simulink model "PPRZ2l"  (R2016b)
settings: Solver=VariableStepAuto  StartTime=0.0  StopTime=10.0  RelTol=1e-3
settings Model: Creator=kkajak  LastModifiedBy=Karl

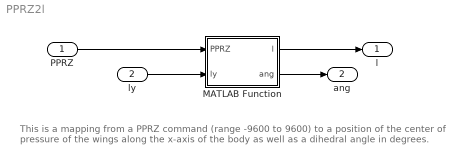
== system PPRZ2l ==
  note: This is a mapping from a PPRZ command (range -9600 to 9600) to a position of the center
      | of pressure of the wings along the x-axis of the body as well as a dihedral angle in degrees.
  PPRZ : Inport
  "ly " : Inport  Port=2
  MATLAB Function : MATLAB Function  TreatAsAtomicUnit=on
  l : Outport
  ang : Outport  Port=2
  wires:
  PPRZ/1 -> MATLAB Function/1(PPRZ)
  "ly "/1 -> MATLAB Function/2(ly)
  MATLAB Function/1(l) -> l/1
  MATLAB Function/2(ang) -> ang/1

== matlab function PPRZ2l/MATLAB Function ==
  data: PPRZ input; l output; ly input; ang output
function [l,ang] = fcn(PPRZ,ly)

ang = -PPRZ/9600*18;
l = ly*sind(ang);
